simulink model "payload_3dof"  (R2024b)
settings: configuration reference "prj_default_config" (kept outside this file)
undefined symbols (not defined in the file or in its folder): CONTROL_PARAM
libraries: matrix_library x3, mqlib x1
settings Model: Creator=yangyu  LastModifiedBy=yangyu
settings ConfigSetRef: SourceName=prj_default_config  SourceLocation=Base Workspace

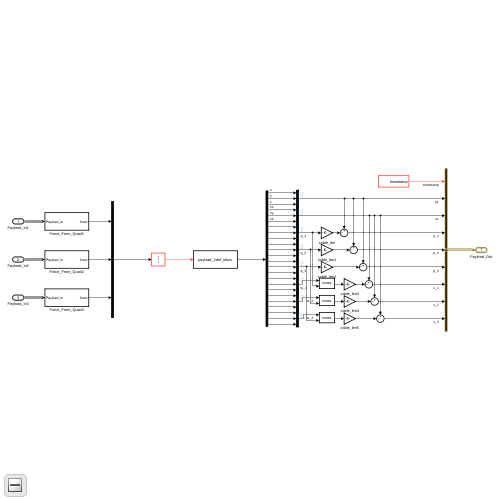
[thumbnail: Simulink's stored preview of the top-level diagram]
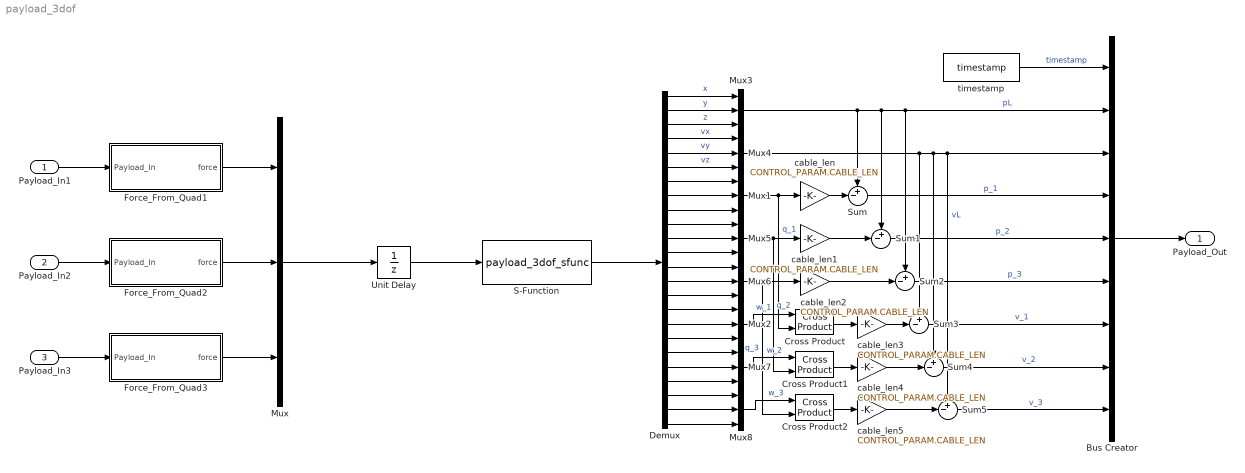
== system payload_3dof ==
  Payload_In1 : Inport  OutDataTypeStr=Bus: Payload_In_Bus
  Payload_In2 : Inport  Port=2  OutDataTypeStr=Bus: Payload_In_Bus
  Payload_In3 : Inport  Port=3  OutDataTypeStr=Bus: Payload_In_Bus
  Bus Creator : BusCreator  Inputs=9  OutDataTypeStr=Bus: Payload_Out_Bus
  Cross Product : matrix_library/Cross Product
  Cross Product1 : matrix_library/Cross Product
  Cross Product2 : matrix_library/Cross Product
  Demux : Demux  Outputs=24
  Force_From_Quad1 : Subsystem
  Force_From_Quad2 : Subsystem
  Force_From_Quad3 : Subsystem
  Mux{,1..8} (9 alike) : Mux  Inputs=3
  S-Function : S-Function  FunctionName=payload_3dof_sfunc  SFunctionDeploymentMode=off  EnableBusSupport=off
  Sum{,1..5} (6 alike) : Sum  Inputs=+-|
  Unit Delay : UnitDelay  SampleTime=-1  HasFrameUpgradeWarning=on
  cable_len{,1..5} (6 alike) : Gain  Gain=CONTROL_PARAM.CABLE_LEN
  timestamp : mqlib/timestamp
  Payload_Out : Outport  OutDataTypeStr=Bus: Payload_Out_Bus
  wires:
  S-Function/1 -> Demux/1
  Demux/1 -> Mux3/1  "x"
  Demux/2 -> Mux3/2  "y"
  Demux/3 -> Mux3/3  "z"
  Force_From_Quad1/1(force) -> Mux/1
  Demux/4 -> Mux4/1  "vx"
  Demux/5 -> Mux4/2  "vy"
  Demux/6 -> Mux4/3  "vz"
  Force_From_Quad2/1(force) -> Mux/2
  Force_From_Quad3/1(force) -> Mux/3
  Payload_In1/1 -> Force_From_Quad1/1(Payload_In)
  Payload_In2/1 -> Force_From_Quad2/1(Payload_In)
  Payload_In3/1 -> Force_From_Quad3/1(Payload_In)
  timestamp/1 -> Bus Creator/1  "timestamp"
  Bus Creator/1 -> Payload_Out/1
  Mux/1 -> Unit Delay/1
  Unit Delay/1 -> S-Function/1
  Mux2/1 -> Cross Product/1  "w_1"
  Mux5/1 -> Cross Product1/2, cable_len1/1  "q_2"
  Mux6/1 -> Cross Product2/2, cable_len2/1  "q_3"
  Mux8/1 -> Cross Product2/1  "w_3"
  Mux1/1 -> cable_len/1, Cross Product/2  "q_1"
  Mux7/1 -> Cross Product1/1  "w_2"
  Demux/7 -> Mux1/1
  Demux/8 -> Mux1/2
  Demux/9 -> Mux1/3
  Demux/10 -> Mux5/1
  Demux/11 -> Mux5/2
  Demux/12 -> Mux5/3
  Demux/13 -> Mux6/1
  Demux/14 -> Mux6/2
  Demux/15 -> Mux6/3
  Demux/16 -> Mux2/1
  Demux/17 -> Mux2/2
  Demux/18 -> Mux2/3
  Demux/19 -> Mux7/1
  Demux/20 -> Mux7/2
  Demux/21 -> Mux7/3
  Demux/22 -> Mux8/1
  Demux/23 -> Mux8/2
  Demux/24 -> Mux8/3
  cable_len/1 -> Sum/2
  cable_len1/1 -> Sum1/2
  cable_len2/1 -> Sum2/2
  Sum/1 -> Bus Creator/4  "p_1"
  Sum1/1 -> Bus Creator/5  "p_2"
  Sum2/1 -> Bus Creator/6  "p_3"
  Cross Product/1 -> cable_len3/1
  cable_len3/1 -> Sum3/2
  Sum3/1 -> Bus Creator/7  "v_1"
  Cross Product1/1 -> cable_len4/1
  cable_len4/1 -> Sum4/2
  Sum4/1 -> Bus Creator/8  "v_2"
  Cross Product2/1 -> cable_len5/1
  cable_len5/1 -> Sum5/2
  Sum5/1 -> Bus Creator/9  "v_3"
  Mux3/1 -> Sum/1, Sum1/1, Bus Creator/2, Sum2/1  "pL"
  Mux4/1 -> Bus Creator/3, Sum5/1, Sum4/1, Sum3/1  "vL"

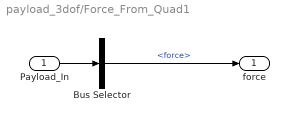
== system payload_3dof/Force_From_Quad1 ==
  Payload_In : Inport
  Bus Selector : BusSelector  OutputSignals=force
  force : Outport
  wires:
  Payload_In/1 -> Bus Selector/1
  Bus Selector/1 -> force/1  "<force>"

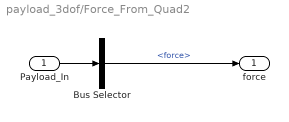
== system payload_3dof/Force_From_Quad2 ==
  Payload_In : Inport
  Bus Selector : BusSelector  OutputSignals=force
  force : Outport
  wires:
  Bus Selector/1 -> force/1  "<force>"
  Payload_In/1 -> Bus Selector/1

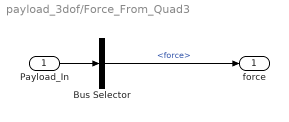
== system payload_3dof/Force_From_Quad3 ==
  Payload_In : Inport
  Bus Selector : BusSelector  OutputSignals=force
  force : Outport
  wires:
  Payload_In/1 -> Bus Selector/1
  Bus Selector/1 -> force/1  "<force>"
